simulink model "ClassifyHumanActivityByIncrementalLearning"  (R2022a)
settings: Solver=FixedStepAuto  StartTime=0.0  StopTime=10340  RelTol=1e-3
libraries: dspsrcs4 x2, simulink x1
settings Model: SnapshotBufferSize=100  SnapshotInterval=100  Creator=tyoshida  LastModifiedBy=tyoshida
settings DebuggingCC: UnconnectedInputMsg=warning  UnconnectedOutputMsg=warning  UnconnectedLineMsg=warning
settings RTWCC: DLArmComputeVersion=19.05

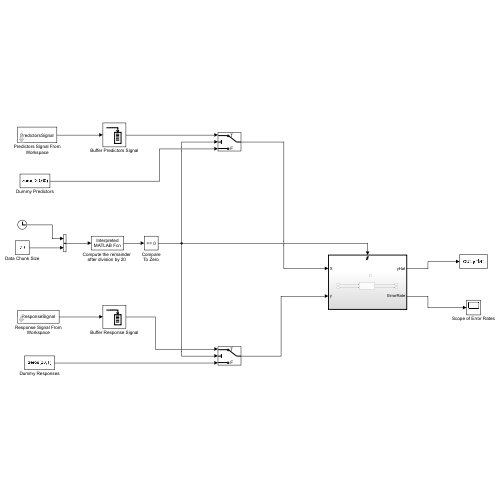
[thumbnail: Simulink's stored preview of the top-level diagram]
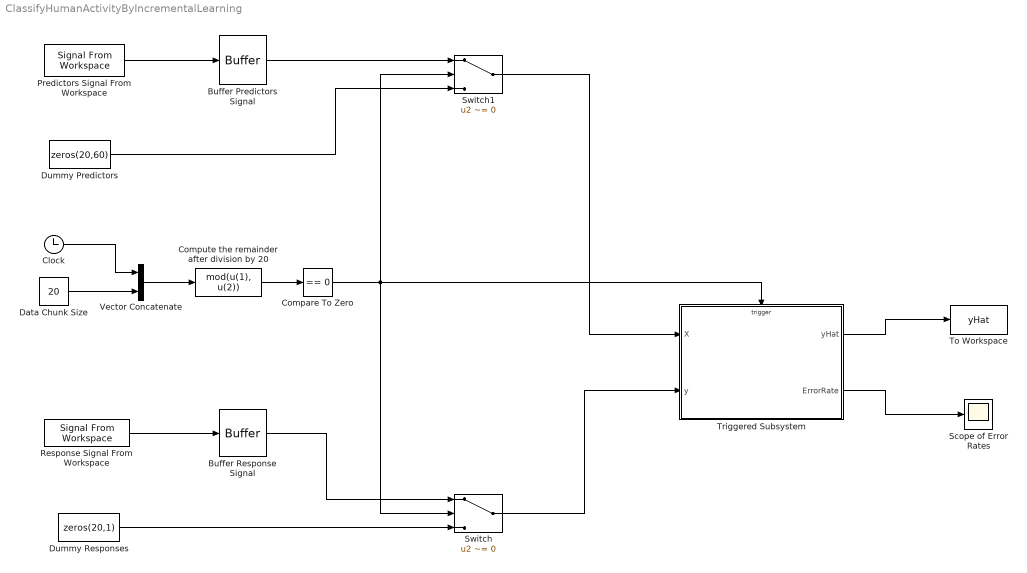
== system ClassifyHumanActivityByIncrementalLearning ==
  Buffer Predictors Signal : Buffer  N=20  OutputFrames=off
  Buffer Response Signal : Buffer  N=20  OutputFrames=off
  Clock : Clock
  Compare To Zero : simulink/Logic and Bit Operations/Compare To Constant  relop===  const=0  OutDataTypeStr=boolean
  "Compute the remainder after division by 20 " : MATLABFcn  MATLABFcn=mod(u(1), u(2))
  Data Chunk Size : Constant  Value=20
  Dummy Predictors : Constant  Value=zeros(20,60)
  Dummy Responses : Constant  Value=zeros(20,1)
  Predictors Signal From Workspace : dspsrcs4/Signal From Workspace  X=PredictorsSignal  Ts=1  nsamps=1  OutputAfterFinalValue=Setting to zero  ignoreOrWarnInputAndFrameLengths=off  OutputFrames=off
  Response Signal From Workspace : dspsrcs4/Signal From Workspace  X=ResponseSignal  Ts=1  nsamps=1  OutputAfterFinalValue=Setting to zero  ignoreOrWarnInputAndFrameLengths=off  OutputFrames=on
  Scope of Error Rates : Scope
  Switch : Switch  Criteria=u2 ~= 0  SaturateOnIntegerOverflow=off  InputSameDT=off
  Switch1 : Switch  Criteria=u2 ~= 0  SaturateOnIntegerOverflow=off  InputSameDT=off
  To Workspace : ToWorkspace  VariableName=yHat  SaveFormat=Timeseries  SampleTime=-1
  Triggered Subsystem : Subsystem  TreatAsAtomicUnit=on
  Vector Concatenate : Concatenate
  wires:
  "Compute the remainder after division by 20 "/1 -> Compare To Zero/1
  Triggered Subsystem/2(ErrorRate) -> Scope of Error Rates/1
  Triggered Subsystem/1(yHat) -> To Workspace/1
  Predictors Signal From Workspace/1 -> Buffer Predictors Signal/1
  Switch1/1 -> Triggered Subsystem/1(X)
  Dummy Predictors/1 -> Switch1/3
  Compare To Zero/1 -> Triggered Subsystem/Trigger, Switch/2, Switch1/2
  Dummy Responses/1 -> Switch/3
  Vector Concatenate/1 -> "Compute the remainder after division by 20 "/1
  Response Signal From Workspace/1 -> Buffer Response Signal/1
  Data Chunk Size/1 -> Vector Concatenate/2
  Switch/1 -> Triggered Subsystem/2(y)
  Buffer Predictors Signal/1 -> Switch1/1
  Clock/1 -> Vector Concatenate/1
  Buffer Response Signal/1 -> Switch/1

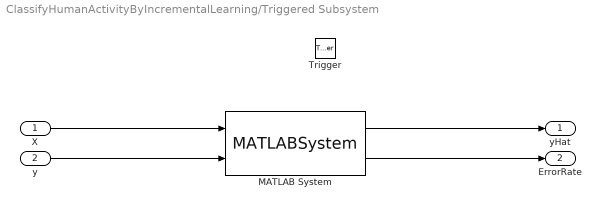
== system ClassifyHumanActivityByIncrementalLearning/Triggered Subsystem ==
  X : Inport
  y : Inport  Port=2
  Trigger : TriggerPort  VariantControl=(inherit)
  MATLAB System : MATLABSystem  System=mySysObj  ChunkSize=20  SimulateUsing=Interpreted execution
      mask Type: mySysObj
      mask Display:
      | disp(['Incremental' char(10) 'Classifier' char(10) '(Naive Bayes)']);
      | port_label('input',1,'X');
      | port_label('input',2,'y');
      | port_label('output',1,'yHat');
      | port_label('output',2,'eRate');
  yHat : Outport
  ErrorRate : Outport  Port=2
  wires:
  X/1 -> MATLAB System/1
  MATLAB System/1 -> yHat/1
  y/1 -> MATLAB System/2
  MATLAB System/2 -> ErrorRate/1
